simulink library "T_Ground_Undisturbed"  (R2013b)
settings: Solver=ode45  StartTime=0.0  StopTime=10.0  RelTol=1e-3
settings Model: Creator=drhf  LastModifiedBy=drhf

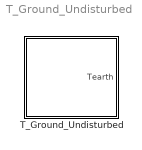
== system T_Ground_Undisturbed ==
  T_Ground_Undisturbed : Subsystem  mask(Undisturbed ground temperature){Tmeanoutside=0, deltathetae=10, tshift=0, cond_ground=1, rhocp=1000*2000, hh=10, znodes=10}
      mask prompts: Tmeanoutside "mean outside temperature over one year [°C]"; deltathetae "amplitude of monthly outside temperatures [°C]"; tshift "time shift where external temperature sine-curve shows a minimum [h]"; cond_ground "soil thermal conductivity in W/m/K"; rhocp "soil heat capacity per Volume in J/m³/K"; hh "depth z in m"; znodes "number of nodes"
      mask help:
      | The temperature of the undisturbed ground Tg is caclulated for a number of equidistant nodes from the surface down to a depth z.
      |
      | Tg = Tavg - dTavg * exp(-z/dg) * cos(2*pi*(t-ts)/t0 - z/dg) + G*z
      |
      | penetration depth : dg = sqrt(t0*cond/(pi*dens*cp))
      |
      | cond  : thermal conductivity of the ground in W/m/K
      | cp    : heat capacity of the ground in J/kg/K
      | dens  : density of the ground in kg/m³
      | G     : temperature increase in the depth (= 0.03 K/m)
      | t     : time of the year in seconds
      | t0    : total seconds of one year (= 3600*24*365)
      | ts    : time in seconds where the ambient temperature curve shows a minimum
      | Tavg  : annual mean ambient temperature
      | dTavg : annual amplitude of the ambient temperature
      | z     : depth in meters
      |
      | The equation is based on approaches presented in the literature for seasonal temperature variations in the earth’s crust (Baehr & Stephan 2006; Wesselak & Schabbach 2009), neglecting the influence of the heat transfer resistance from the ambient air to the surface of the ground (i.e. u_surf =):
      mask init:
      | %thermische eindringtiefe
      | delta_grd = sqrt((8760*3600*cond_ground)/(pi*rhocp));
      | 
      | % height vector
      | z = [0:hh/znodes:hh];
      mask Help: web(fullfile(path_carnot('help'),'T_Ground_Undisturbed.html'),'-helpbrowser')
      mask Display: plot(0,0,100,100,[90,10],[90,90],[50,50],[-0,90],[49,48,46,44,41,34,25,15],[-0,20,40,50,60,70,80,90],[52,54,56,58,61,67,76,85],[-0,20,40,50,60,70,80,90],[50,49,49,48,48,48,50,54,60],[-0,20,30,40,50,60,70,80,90],[50,51,51,52,52,50,48,43,35],[0,20,30,40,50,60,70,80,90])

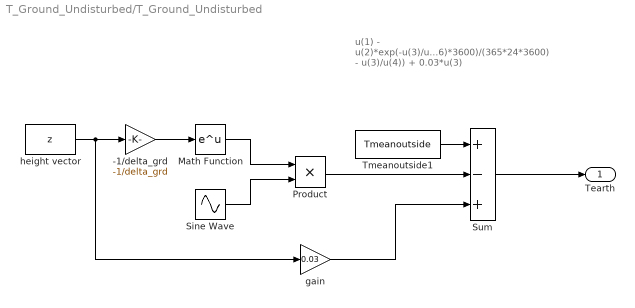
== system T_Ground_Undisturbed/T_Ground_Undisturbed ==
  note: u(1) - u(2)*exp(-u(3)/u(4))*cos(2*pi*(u(5)-u(6)*3600)/(365*24*3600) - u(3)/u(4)) + 0.03*u(3)
  -1/delta_grd : Gain  Gain=-1/delta_grd
  Math Function : Math  SaturateOnIntegerOverflow=on
  Product : Product  RndMeth=Zero
  Sine Wave : Sin  Amplitude=deltathetae  Frequency=2*pi/(365*24*3600)  Phase=pi/2 - 2*pi*tshift/(365*24) - z/delta_grd  SampleTime=0
  Sum : Sum  Inputs=+-+
  Tmeanoutside1 : Constant  Value=Tmeanoutside
  gain : Gain  Gain=0.03
  height vector : Constant  Value=z
  Tearth : Outport
  wires:
  gain/1 -> Sum/3
  height vector/1 -> gain/1, -1/delta_grd/1
  -1/delta_grd/1 -> Math Function/1
  Math Function/1 -> Product/1
  Sine Wave/1 -> Product/2
  Product/1 -> Sum/2
  Sum/1 -> Tearth/1
  Tmeanoutside1/1 -> Sum/1
